simulink library "Ta_Library"  (R2019b)
settings: Solver=VariableStepAuto  StartTime=0.0  StopTime=10.0  RelTol=1e-3
undefined symbols (not defined in the file): AEBSFunctionLib, StateDelayAbortion, TargetClassification
libraries: Mylibrary x5, simulink x1
(part 3 of 3)

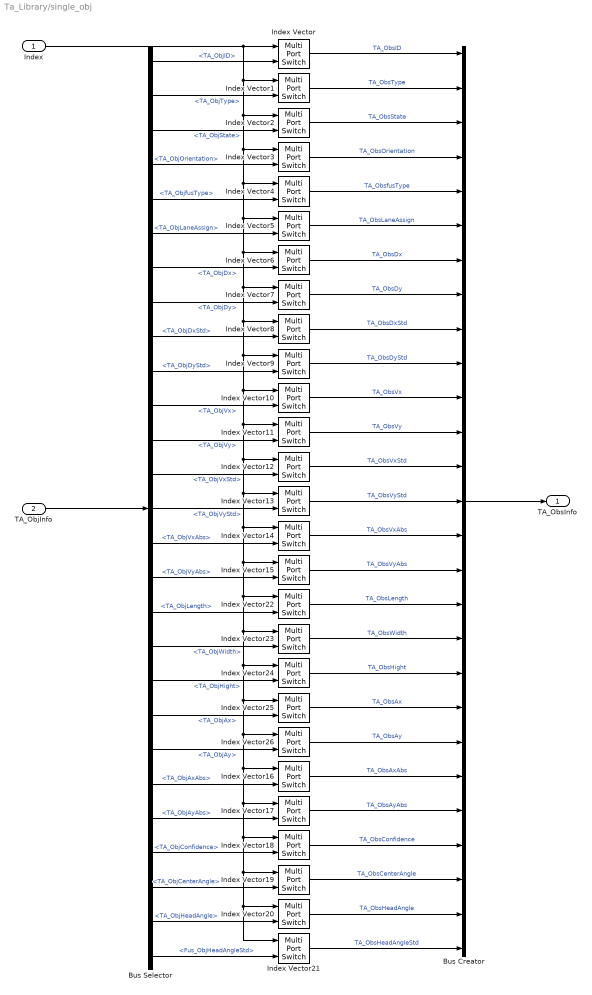
== system Ta_Library/single_obj ==
  Index : Inport
  TA_ObjInfo : Inport  Port=2
  Bus Creator : BusCreator  Inputs=27
  Bus Selector : BusSelector  OutputSignals=TA_ObjID,TA_ObjType,TA_ObjState,TA_ObjOrientation,TA_ObjfusType,TA_ObjLaneAssign,TA_ObjDx,TA_ObjDy,TA_ObjDxStd,TA_ObjDyStd,TA_ObjVx,TA_ObjVy,TA_ObjVxStd,TA_ObjVyStd,TA_ObjVxAbs,TA_ObjVyAbs,TA_ObjLength,TA_ObjWidth,TA_ObjHight,TA_ObjAx,TA_ObjAy,TA_ObjAxAbs,TA_ObjAyAbs,TA_ObjConfidence,TA_ObjCenterAngle,TA_ObjHeadAngle,Fus_ObjHeadAngleStd
  Index Vector{,1..26} (27 alike) : MultiPortSwitch  Inputs=1
  TA_ObsInfo : Outport
  wires:
  TA_ObjInfo/1 -> Bus Selector/1
  Bus Selector/1 -> Index Vector/2  "<TA_ObjID>"
  Index/1 -> Index Vector21/1, Index Vector20/1, Index Vector19/1, Index Vector18/1, Index Vector17/1, Index Vector16/1, Index Vector26/1, Index Vector25/1, Index Vector24/1, Index Vector23/1, Index Vector22/1, Index Vector15/1, Index Vector14/1, Index Vector13/1, Index Vector12/1, Index Vector11/1, Index Vector10/1, Index Vector9/1, Index Vector8/1, Index Vector7/1, Index Vector6/1, Index Vector5/1, Index Vector4/1, Index Vector3/1, Index Vector2/1, Index Vector1/1, Index Vector/1
  Bus Selector/2 -> Index Vector1/2  "<TA_ObjType>"
  Bus Selector/3 -> Index Vector2/2  "<TA_ObjState>"
  Bus Selector/4 -> Index Vector3/2  "<TA_ObjOrientation>"
  Bus Selector/5 -> Index Vector4/2  "<TA_ObjfusType>"
  Bus Selector/6 -> Index Vector5/2  "<TA_ObjLaneAssign>"
  Bus Selector/7 -> Index Vector6/2  "<TA_ObjDx>"
  Bus Selector/8 -> Index Vector7/2  "<TA_ObjDy>"
  Bus Selector/9 -> Index Vector8/2  "<TA_ObjDxStd>"
  Bus Selector/10 -> Index Vector9/2  "<TA_ObjDyStd>"
  Bus Selector/11 -> Index Vector10/2  "<TA_ObjVx>"
  Bus Selector/12 -> Index Vector11/2  "<TA_ObjVy>"
  Bus Selector/13 -> Index Vector12/2  "<TA_ObjVxStd>"
  Bus Selector/14 -> Index Vector13/2  "<TA_ObjVyStd>"
  Bus Selector/15 -> Index Vector14/2  "<TA_ObjVxAbs>"
  Bus Selector/16 -> Index Vector15/2  "<TA_ObjVyAbs>"
  Bus Selector/17 -> Index Vector22/2  "<TA_ObjLength>"
  Bus Selector/18 -> Index Vector23/2  "<TA_ObjWidth>"
  Bus Selector/19 -> Index Vector24/2  "<TA_ObjHight>"
  Bus Selector/20 -> Index Vector25/2  "<TA_ObjAx>"
  Bus Selector/21 -> Index Vector26/2  "<TA_ObjAy>"
  Bus Selector/22 -> Index Vector16/2  "<TA_ObjAxAbs>"
  Bus Selector/23 -> Index Vector17/2  "<TA_ObjAyAbs>"
  Bus Selector/24 -> Index Vector18/2  "<TA_ObjConfidence>"
  Bus Selector/25 -> Index Vector19/2  "<TA_ObjCenterAngle>"
  Bus Selector/26 -> Index Vector20/2  "<TA_ObjHeadAngle>"
  Bus Selector/27 -> Index Vector21/2  "<Fus_ObjHeadAngleStd>"
  Index Vector15/1 -> Bus Creator/16  "TA_ObsVyAbs"
  Index Vector14/1 -> Bus Creator/15  "TA_ObsVxAbs"
  Index Vector22/1 -> Bus Creator/17  "TA_ObsLength"
  Index Vector13/1 -> Bus Creator/14  "TA_ObsVyStd"
  Index Vector23/1 -> Bus Creator/18  "TA_ObsWidth"
  Index Vector12/1 -> Bus Creator/13  "TA_ObsVxStd"
  Index Vector24/1 -> Bus Creator/19  "TA_ObsHight"
  Index Vector11/1 -> Bus Creator/12  "TA_ObsVy"
  Index Vector25/1 -> Bus Creator/20  "TA_ObsAx"
  Index Vector10/1 -> Bus Creator/11  "TA_ObsVx"
  Index Vector26/1 -> Bus Creator/21  "TA_ObsAy"
  Index Vector9/1 -> Bus Creator/10  "TA_ObsDyStd"
  Index Vector16/1 -> Bus Creator/22  "TA_ObsAxAbs"
  Index Vector8/1 -> Bus Creator/9  "TA_ObsDxStd"
  Index Vector17/1 -> Bus Creator/23  "TA_ObsAyAbs"
  Index Vector7/1 -> Bus Creator/8  "TA_ObsDy"
  Index Vector18/1 -> Bus Creator/24  "TA_ObsConfidence"
  Index Vector6/1 -> Bus Creator/7  "TA_ObsDx"
  Index Vector19/1 -> Bus Creator/25  "TA_ObsCenterAngle"
  Index Vector5/1 -> Bus Creator/6  "TA_ObsLaneAssign"
  Index Vector20/1 -> Bus Creator/26  "TA_ObsHeadAngle"
  Index Vector4/1 -> Bus Creator/5  "TA_ObsfusType"
  Index Vector21/1 -> Bus Creator/27  "TA_ObsHeadAngleStd"
  Index Vector3/1 -> Bus Creator/4  "TA_ObsOrientation"
  Index Vector2/1 -> Bus Creator/3  "TA_ObsState"
  Index Vector1/1 -> Bus Creator/2  "TA_ObsType"
  Index Vector/1 -> Bus Creator/1  "TA_ObsID"
  Bus Creator/1 -> TA_ObsInfo/1

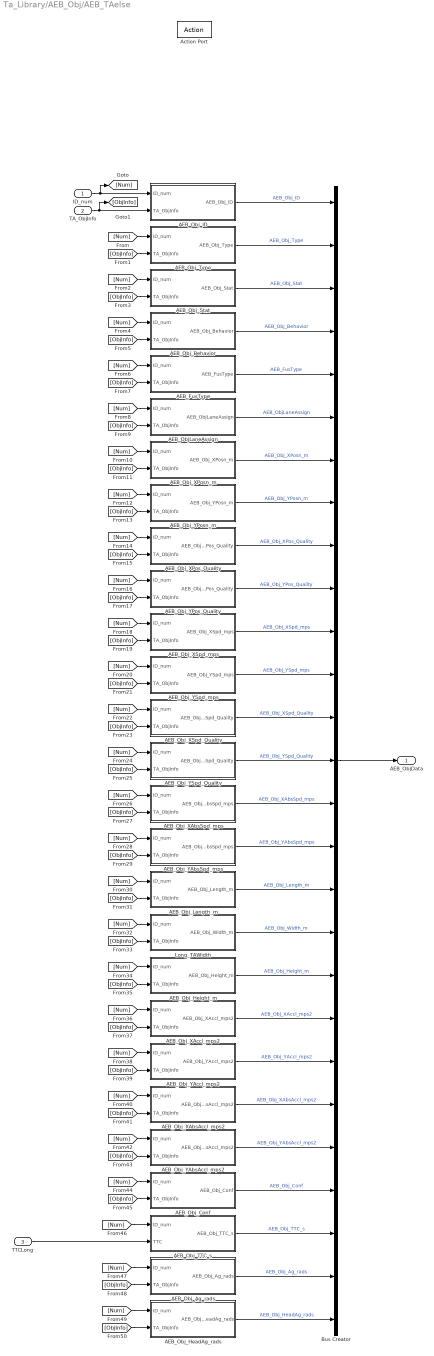
== system Ta_Library/AEB_Obj/AEB_TAelse ==
  ID_num : Inport
  TA_ObjInfo : Inport  Port=2
  TTCLong : Inport  Port=3
  Action Port : ActionPort
  AEB_FusType : Subsystem
  AEB_ObjLaneAssign : Subsystem
  AEB_Obj_Ag_rads : Subsystem
  AEB_Obj_Behavior : Subsystem
  AEB_Obj_Conf : Subsystem
  AEB_Obj_HeadAg_rads : Subsystem
  AEB_Obj_Height_m : Subsystem
  AEB_Obj_ID : Subsystem
  AEB_Obj_Length_m : Subsystem
  AEB_Obj_Stat : Subsystem
  AEB_Obj_TTC_s : Subsystem
  AEB_Obj_Type : Subsystem
  AEB_Obj_XAbsAccl_mps2 : Subsystem
  AEB_Obj_XAbsSpd_mps : Subsystem
  AEB_Obj_XAccl_mps2 : Subsystem
  AEB_Obj_XPos_Quality : Subsystem
  AEB_Obj_XPosn_m : Subsystem
  AEB_Obj_XSpd_Quality : Subsystem
  AEB_Obj_XSpd_mps : Subsystem
  AEB_Obj_YAbsAccl_mps2 : Subsystem
  AEB_Obj_YAbsSpd_mps : Subsystem
  AEB_Obj_YAccl_mps2 : Subsystem
  AEB_Obj_YPos_Quality : Subsystem
  AEB_Obj_YPosn_m : Subsystem
  AEB_Obj_YSpd_Quality : Subsystem
  AEB_Obj_YSpd_mps : Subsystem
  Bus Creator : BusCreator  Inputs=27
  Long_TAWidth : Subsystem
  AEB_ObjData : Outport
  wires:
  Long_TAWidth/1(AEB_Obj_Width_m) -> Bus Creator/18  "AEB_Obj_Width_m"
  AEB_Obj_YSpd_mps/1(AEB_Obj_YSpd_mps) -> Bus Creator/12  "AEB_Obj_YSpd_mps"
  AEB_Obj_XSpd_Quality/1(AEB_Obj_XSpd_Quality) -> Bus Creator/13  "AEB_Obj_XSpd_Quality"
  AEB_Obj_XAbsSpd_mps/1(AEB_Obj_XAbsSpd_mps) -> Bus Creator/15  "AEB_Obj_XAbsSpd_mps"
  AEB_Obj_YSpd_Quality/1(AEB_Obj_YSpd_Quality) -> Bus Creator/14  "AEB_Obj_YSpd_Quality"
  AEB_FusType/1(AEB_FusType) -> Bus Creator/5  "AEB_FusType"
  AEB_ObjLaneAssign/1(AEB_ObjLaneAssign) -> Bus Creator/6  "AEB_ObjLaneAssign"
  AEB_Obj_Length_m/1(AEB_Obj_Length_m) -> Bus Creator/17  "AEB_Obj_Length_m"
  AEB_Obj_XSpd_mps/1(AEB_Obj_XSpd_mps) -> Bus Creator/11  "AEB_Obj_XSpd_mps"
  AEB_Obj_YPos_Quality/1(AEB_Obj_YPos_Quality) -> Bus Creator/10  "AEB_Obj_YPos_Quality"
  AEB_Obj_Type/1(AEB_Obj_Type) -> Bus Creator/2  "AEB_Obj_Type"
  AEB_Obj_YAbsSpd_mps/1(AEB_Obj_YAbsSpd_mps) -> Bus Creator/16  "AEB_Obj_YAbsSpd_mps"
  AEB_Obj_ID/1(AEB_Obj_ID) -> Bus Creator/1  "AEB_Obj_ID"
  AEB_Obj_XPos_Quality/1(AEB_Obj_XPos_Quality) -> Bus Creator/9  "AEB_Obj_XPos_Quality"
  AEB_Obj_Behavior/1(AEB_Obj_Behavior) -> Bus Creator/4  "AEB_Obj_Behavior"
  AEB_Obj_Stat/1(AEB_Obj_Stat) -> Bus Creator/3  "AEB_Obj_Stat"
  AEB_Obj_YPosn_m/1(AEB_Obj_YPosn_m) -> Bus Creator/8  "AEB_Obj_YPosn_m"
  Bus Creator/1 -> AEB_ObjData/1
  AEB_Obj_XPosn_m/1(AEB_Obj_XPosn_m) -> Bus Creator/7  "AEB_Obj_XPosn_m"
  ID_num/1 -> AEB_Obj_ID/1(ID_num), [Num]
  TA_ObjInfo/1 -> [ObjInfo], AEB_Obj_ID/2(TA_ObjInfo)
  [Num] -> AEB_Obj_Type/1(ID_num)
  [ObjInfo] -> AEB_Obj_Type/2(TA_ObjInfo)
  [Num] -> AEB_Obj_Stat/1(ID_num)
  [ObjInfo] -> AEB_Obj_Stat/2(TA_ObjInfo)
  [ObjInfo] -> AEB_Obj_Behavior/2(TA_ObjInfo)
  [Num] -> AEB_Obj_Behavior/1(ID_num)
  [Num] -> AEB_FusType/1(ID_num)
  [ObjInfo] -> AEB_FusType/2(TA_ObjInfo)
  [ObjInfo] -> AEB_ObjLaneAssign/2(TA_ObjInfo)
  [Num] -> AEB_ObjLaneAssign/1(ID_num)
  [Num] -> AEB_Obj_XPosn_m/1(ID_num)
  [ObjInfo] -> AEB_Obj_XPosn_m/2(TA_ObjInfo)
  [ObjInfo] -> AEB_Obj_YPosn_m/2(TA_ObjInfo)
  [Num] -> AEB_Obj_YPosn_m/1(ID_num)
  [Num] -> AEB_Obj_XPos_Quality/1(ID_num)
  [ObjInfo] -> AEB_Obj_XPos_Quality/2(TA_ObjInfo)
  [ObjInfo] -> AEB_Obj_YPos_Quality/2(TA_ObjInfo)
  [Num] -> AEB_Obj_YPos_Quality/1(ID_num)
  [Num] -> AEB_Obj_XSpd_mps/1(ID_num)
  [ObjInfo] -> AEB_Obj_XSpd_mps/2(TA_ObjInfo)
  [ObjInfo] -> AEB_Obj_YSpd_mps/2(TA_ObjInfo)
  [Num] -> AEB_Obj_YSpd_mps/1(ID_num)
  [Num] -> AEB_Obj_XSpd_Quality/1(ID_num)
  [ObjInfo] -> AEB_Obj_XSpd_Quality/2(TA_ObjInfo)
  [ObjInfo] -> AEB_Obj_YSpd_Quality/2(TA_ObjInfo)
  [Num] -> AEB_Obj_YSpd_Quality/1(ID_num)
  [Num] -> AEB_Obj_XAbsSpd_mps/1(ID_num)
  [ObjInfo] -> AEB_Obj_XAbsSpd_mps/2(TA_ObjInfo)
  [ObjInfo] -> AEB_Obj_YAbsSpd_mps/2(TA_ObjInfo)
  [Num] -> AEB_Obj_YAbsSpd_mps/1(ID_num)
  [Num] -> AEB_Obj_Length_m/1(ID_num)
  [ObjInfo] -> AEB_Obj_Length_m/2(TA_ObjInfo)
  [ObjInfo] -> Long_TAWidth/2(TA_ObjInfo)
  [Num] -> Long_TAWidth/1(ID_num)
  [Num] -> AEB_Obj_Height_m/1(ID_num)
  [ObjInfo] -> AEB_Obj_Height_m/2(TA_ObjInfo)
  AEB_Obj_Height_m/1(AEB_Obj_Height_m) -> Bus Creator/19  "AEB_Obj_Height_m"
  [ObjInfo] -> AEB_Obj_XAccl_mps2/2(TA_ObjInfo)
  [Num] -> AEB_Obj_XAccl_mps2/1(ID_num)
  [Num] -> AEB_Obj_YAccl_mps2/1(ID_num)
  [ObjInfo] -> AEB_Obj_YAccl_mps2/2(TA_ObjInfo)
  [ObjInfo] -> AEB_Obj_YAbsAccl_mps2/2(TA_ObjInfo)
  [Num] -> AEB_Obj_YAbsAccl_mps2/1(ID_num)
  [Num] -> AEB_Obj_XAbsAccl_mps2/1(ID_num)
  [ObjInfo] -> AEB_Obj_XAbsAccl_mps2/2(TA_ObjInfo)
  [Num] -> AEB_Obj_Conf/1(ID_num)
  [ObjInfo] -> AEB_Obj_Conf/2(TA_ObjInfo)
  [Num] -> AEB_Obj_TTC_s/1(ID_num)
  TTCLong/1 -> AEB_Obj_TTC_s/2(TTC)
  [ObjInfo] -> AEB_Obj_Ag_rads/2(TA_ObjInfo)
  [Num] -> AEB_Obj_Ag_rads/1(ID_num)
  [Num] -> AEB_Obj_HeadAg_rads/1(ID_num)
  [ObjInfo] -> AEB_Obj_HeadAg_rads/2(TA_ObjInfo)
  AEB_Obj_XAccl_mps2/1(AEB_Obj_XAccl_mps2) -> Bus Creator/20  "AEB_Obj_XAccl_mps2"
  AEB_Obj_YAccl_mps2/1(AEB_Obj_YAccl_mps2) -> Bus Creator/21  "AEB_Obj_YAccl_mps2"
  AEB_Obj_XAbsAccl_mps2/1(AEB_Obj_XAbsAccl_mps2) -> Bus Creator/22  "AEB_Obj_XAbsAccl_mps2"
  AEB_Obj_YAbsAccl_mps2/1(AEB_Obj_YAbsAccl_mps2) -> Bus Creator/23  "AEB_Obj_YAbsAccl_mps2"
  AEB_Obj_Conf/1(AEB_Obj_Conf) -> Bus Creator/24  "AEB_Obj_Conf"
  AEB_Obj_TTC_s/1(AEB_Obj_TTC_s) -> Bus Creator/25  "AEB_Obj_TTC_s"
  AEB_Obj_Ag_rads/1(AEB_Obj_Ag_rads) -> Bus Creator/26  "AEB_Obj_Ag_rads"
  AEB_Obj_HeadAg_rads/1(AEB_Obj_HeadAg_rads) -> Bus Creator/27  "AEB_Obj_HeadAg_rads"

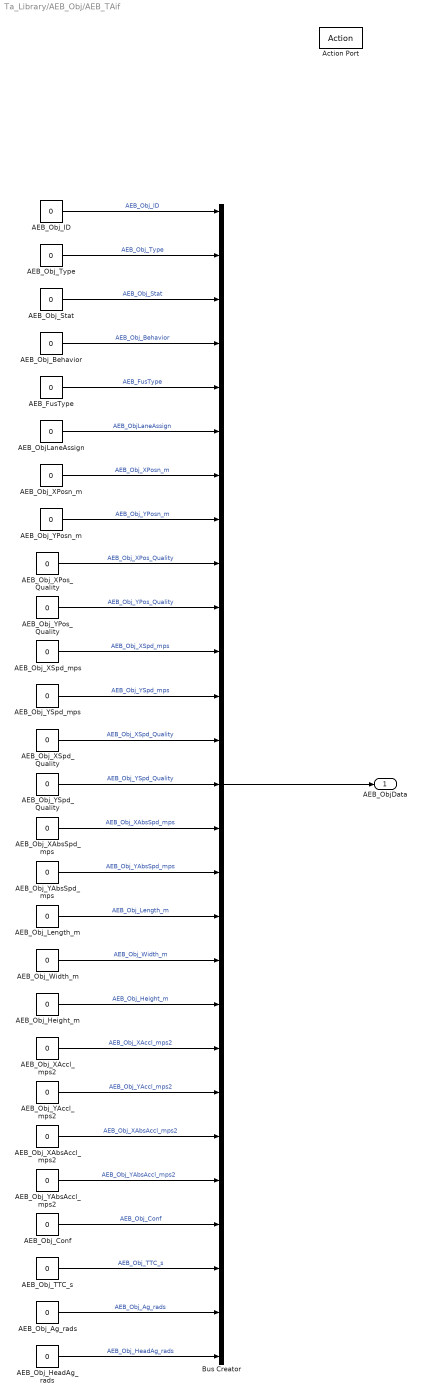
== system Ta_Library/AEB_Obj/AEB_TAif ==
  Action Port : ActionPort
  AEB_FusType : Constant  Value=0  OutDataTypeStr=uint8
  AEB_ObjLaneAssign : Constant  Value=0  OutDataTypeStr=uint8
  AEB_Obj_Ag_rads : Constant  Value=0  OutDataTypeStr=single
  AEB_Obj_Behavior : Constant  Value=0  OutDataTypeStr=uint8
  AEB_Obj_Conf : Constant  Value=0  OutDataTypeStr=uint8
  AEB_Obj_HeadAg_rads : Constant  Value=0  OutDataTypeStr=single
  AEB_Obj_Height_m : Constant  Value=0  OutDataTypeStr=single
  AEB_Obj_ID : Constant  Value=0  OutDataTypeStr=uint8
  AEB_Obj_Length_m : Constant  Value=0  OutDataTypeStr=single
  AEB_Obj_Stat : Constant  Value=0  OutDataTypeStr=uint8
  AEB_Obj_TTC_s : Constant  Value=0  OutDataTypeStr=single
  AEB_Obj_Type : Constant  Value=0  OutDataTypeStr=uint8
  AEB_Obj_Width_m : Constant  Value=0  OutDataTypeStr=single
  AEB_Obj_XAbsAccl_mps2 : Constant  Value=0  OutDataTypeStr=single
  AEB_Obj_XAbsSpd_mps : Constant  Value=0  OutDataTypeStr=single
  AEB_Obj_XAccl_mps2 : Constant  Value=0  OutDataTypeStr=single
  AEB_Obj_XPos_Quality : Constant  Value=0  OutDataTypeStr=single
  AEB_Obj_XPosn_m : Constant  Value=0  OutDataTypeStr=single
  AEB_Obj_XSpd_Quality : Constant  Value=0  OutDataTypeStr=single
  AEB_Obj_XSpd_mps : Constant  Value=0  OutDataTypeStr=single
  AEB_Obj_YAbsAccl_mps2 : Constant  Value=0  OutDataTypeStr=single
  AEB_Obj_YAbsSpd_mps : Constant  Value=0  OutDataTypeStr=single
  AEB_Obj_YAccl_mps2 : Constant  Value=0  OutDataTypeStr=single
  AEB_Obj_YPos_Quality : Constant  Value=0  OutDataTypeStr=single
  AEB_Obj_YPosn_m : Constant  Value=0  OutDataTypeStr=single
  AEB_Obj_YSpd_Quality : Constant  Value=0  OutDataTypeStr=single
  AEB_Obj_YSpd_mps : Constant  Value=0  OutDataTypeStr=single
  Bus Creator : BusCreator  Inputs=27
  AEB_ObjData : Outport
  wires:
  AEB_Obj_ID/1 -> Bus Creator/1  "AEB_Obj_ID"
  AEB_Obj_Type/1 -> Bus Creator/2  "AEB_Obj_Type"
  AEB_Obj_Stat/1 -> Bus Creator/3  "AEB_Obj_Stat"
  AEB_Obj_Behavior/1 -> Bus Creator/4  "AEB_Obj_Behavior"
  AEB_FusType/1 -> Bus Creator/5  "AEB_FusType"
  AEB_ObjLaneAssign/1 -> Bus Creator/6  "AEB_ObjLaneAssign"
  AEB_Obj_XPosn_m/1 -> Bus Creator/7  "AEB_Obj_XPosn_m"
  AEB_Obj_YPosn_m/1 -> Bus Creator/8  "AEB_Obj_YPosn_m"
  AEB_Obj_XPos_Quality/1 -> Bus Creator/9  "AEB_Obj_XPos_Quality"
  AEB_Obj_YPos_Quality/1 -> Bus Creator/10  "AEB_Obj_YPos_Quality"
  AEB_Obj_XSpd_mps/1 -> Bus Creator/11  "AEB_Obj_XSpd_mps"
  AEB_Obj_YSpd_mps/1 -> Bus Creator/12  "AEB_Obj_YSpd_mps"
  AEB_Obj_XSpd_Quality/1 -> Bus Creator/13  "AEB_Obj_XSpd_Quality"
  AEB_Obj_YSpd_Quality/1 -> Bus Creator/14  "AEB_Obj_YSpd_Quality"
  AEB_Obj_XAbsSpd_mps/1 -> Bus Creator/15  "AEB_Obj_XAbsSpd_mps"
  AEB_Obj_YAbsSpd_mps/1 -> Bus Creator/16  "AEB_Obj_YAbsSpd_mps"
  AEB_Obj_Length_m/1 -> Bus Creator/17  "AEB_Obj_Length_m"
  AEB_Obj_Width_m/1 -> Bus Creator/18  "AEB_Obj_Width_m"
  AEB_Obj_Height_m/1 -> Bus Creator/19  "AEB_Obj_Height_m"
  Bus Creator/1 -> AEB_ObjData/1
  AEB_Obj_XAbsAccl_mps2/1 -> Bus Creator/22  "AEB_Obj_XAbsAccl_mps2"
  AEB_Obj_YAbsAccl_mps2/1 -> Bus Creator/23  "AEB_Obj_YAbsAccl_mps2"
  AEB_Obj_XAccl_mps2/1 -> Bus Creator/20  "AEB_Obj_XAccl_mps2"
  AEB_Obj_TTC_s/1 -> Bus Creator/25  "AEB_Obj_TTC_s"
  AEB_Obj_Ag_rads/1 -> Bus Creator/26  "AEB_Obj_Ag_rads"
  AEB_Obj_HeadAg_rads/1 -> Bus Creator/27  "AEB_Obj_HeadAg_rads"
  AEB_Obj_YAccl_mps2/1 -> Bus Creator/21  "AEB_Obj_YAccl_mps2"
  AEB_Obj_Conf/1 -> Bus Creator/24  "AEB_Obj_Conf"

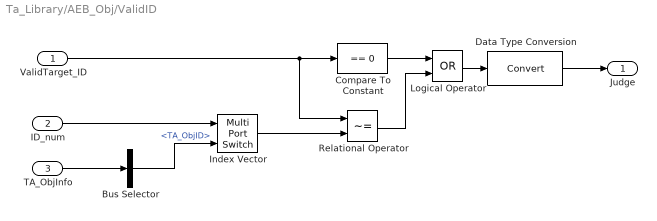
== system Ta_Library/AEB_Obj/ValidID ==
  ValidTarget_ID : Inport
  ID_num : Inport  Port=2
  TA_ObjInfo : Inport  Port=3
  Bus Selector : BusSelector  OutputSignals=TA_ObjInfo.TA_ObjID
  Compare To Constant : simulink/Logic and Bit Operations/Compare To Constant  relop===  const=0  OutDataTypeStr=boolean
  Data Type Conversion : DataTypeConversion
  Index Vector : MultiPortSwitch  Inputs=1
  Logical Operator : Logic  Operator=OR  AllPortsSameDT=off  OutDataTypeStr=boolean
  Relational Operator : RelationalOperator  Operator=~=  OutDataTypeStr=boolean  RndMeth=Simplest
  Judge : Outport
  wires:
  ValidTarget_ID/1 -> Relational Operator/1, Compare To Constant/1
  Data Type Conversion/1 -> Judge/1
  ID_num/1 -> Index Vector/1
  TA_ObjInfo/1 -> Bus Selector/1
  Bus Selector/1 -> Index Vector/2  "<TA_ObjID>"
  Index Vector/1 -> Relational Operator/2
  Compare To Constant/1 -> Logical Operator/1
  Relational Operator/1 -> Logical Operator/2
  Logical Operator/1 -> Data Type Conversion/1

== system Ta_Library/AEB_Obj/AEB_TAelse/AEB_FusType ==
  ID_num : Inport
  TA_ObjInfo : Inport  Port=2
  Bus Selector : BusSelector  OutputSignals=TA_ObjInfo.TA_ObjfusType
  Index Vector : MultiPortSwitch  Inputs=1
  AEB_FusType : Outport
  wires:
  TA_ObjInfo/1 -> Bus Selector/1
  Bus Selector/1 -> Index Vector/2  "<TA_ObjfusType>"
  ID_num/1 -> Index Vector/1
  Index Vector/1 -> AEB_FusType/1

== system Ta_Library/AEB_Obj/AEB_TAelse/AEB_ObjLaneAssign ==
  ID_num : Inport
  TA_ObjInfo : Inport  Port=2
  Bus Selector : BusSelector  OutputSignals=TA_ObjInfo.TA_ObjLaneAssign
  Index Vector : MultiPortSwitch  Inputs=1
  AEB_ObjLaneAssign : Outport
  wires:
  Index Vector/1 -> AEB_ObjLaneAssign/1
  ID_num/1 -> Index Vector/1
  Bus Selector/1 -> Index Vector/2  "<TA_ObjLaneAssign>"
  TA_ObjInfo/1 -> Bus Selector/1

== system Ta_Library/AEB_Obj/AEB_TAelse/AEB_Obj_Ag_rads ==
  ID_num : Inport
  TA_ObjInfo : Inport  Port=2
  Bus Selector : BusSelector  OutputSignals=TA_ObjInfo.TA_ObjCenterAngle
  Index Vector : MultiPortSwitch  Inputs=1
  AEB_Obj_Ag_rads : Outport
  wires:
  Index Vector/1 -> AEB_Obj_Ag_rads/1
  ID_num/1 -> Index Vector/1
  Bus Selector/1 -> Index Vector/2  "<TA_ObjCenterAngle>"
  TA_ObjInfo/1 -> Bus Selector/1

== system Ta_Library/AEB_Obj/AEB_TAelse/AEB_Obj_Behavior ==
  ID_num : Inport
  TA_ObjInfo : Inport  Port=2
  Bus Selector : BusSelector  OutputSignals=TA_ObjInfo.TA_ObjOrientation
  Index Vector : MultiPortSwitch  Inputs=1
  AEB_Obj_Behavior : Outport
  wires:
  Index Vector/1 -> AEB_Obj_Behavior/1
  ID_num/1 -> Index Vector/1
  Bus Selector/1 -> Index Vector/2  "<TA_ObjOrientation>"
  TA_ObjInfo/1 -> Bus Selector/1

== system Ta_Library/AEB_Obj/AEB_TAelse/AEB_Obj_Conf ==
  ID_num : Inport
  TA_ObjInfo : Inport  Port=2
  Bus Selector : BusSelector  OutputSignals=TA_ObjInfo.TA_ObjConfidence
  Index Vector : MultiPortSwitch  Inputs=1
  AEB_Obj_Conf : Outport
  wires:
  TA_ObjInfo/1 -> Bus Selector/1
  Bus Selector/1 -> Index Vector/2  "<TA_ObjConfidence>"
  ID_num/1 -> Index Vector/1
  Index Vector/1 -> AEB_Obj_Conf/1

== system Ta_Library/AEB_Obj/AEB_TAelse/AEB_Obj_HeadAg_rads ==
  ID_num : Inport
  TA_ObjInfo : Inport  Port=2
  Bus Selector : BusSelector  OutputSignals=TA_ObjInfo.TA_ObjHeadAngle
  Index Vector : MultiPortSwitch  Inputs=1
  AEB_Obj_HeadAg_rads : Outport
  wires:
  TA_ObjInfo/1 -> Bus Selector/1
  Bus Selector/1 -> Index Vector/2  "<TA_ObjHeadAngle>"
  ID_num/1 -> Index Vector/1
  Index Vector/1 -> AEB_Obj_HeadAg_rads/1

== system Ta_Library/AEB_Obj/AEB_TAelse/AEB_Obj_Height_m ==
  ID_num : Inport
  TA_ObjInfo : Inport  Port=2
  Bus Selector : BusSelector  OutputSignals=TA_ObjInfo.TA_ObjHight
  Index Vector : MultiPortSwitch  Inputs=1
  AEB_Obj_Height_m : Outport
  wires:
  TA_ObjInfo/1 -> Bus Selector/1
  Bus Selector/1 -> Index Vector/2  "<TA_ObjHight>"
  ID_num/1 -> Index Vector/1
  Index Vector/1 -> AEB_Obj_Height_m/1

== system Ta_Library/AEB_Obj/AEB_TAelse/AEB_Obj_ID ==
  ID_num : Inport
  TA_ObjInfo : Inport  Port=2
  Bus Selector : BusSelector  OutputSignals=TA_ObjInfo.TA_ObjID
  Index Vector : MultiPortSwitch  Inputs=1
  AEB_Obj_ID : Outport
  wires:
  TA_ObjInfo/1 -> Bus Selector/1
  Bus Selector/1 -> Index Vector/2  "<TA_ObjID>"
  ID_num/1 -> Index Vector/1
  Index Vector/1 -> AEB_Obj_ID/1

== system Ta_Library/AEB_Obj/AEB_TAelse/AEB_Obj_Length_m ==
  ID_num : Inport
  TA_ObjInfo : Inport  Port=2
  Bus Selector : BusSelector  OutputSignals=TA_ObjInfo.TA_ObjLength
  Index Vector : MultiPortSwitch  Inputs=1
  AEB_Obj_Length_m : Outport
  wires:
  TA_ObjInfo/1 -> Bus Selector/1
  Bus Selector/1 -> Index Vector/2  "<TA_ObjLength>"
  ID_num/1 -> Index Vector/1
  Index Vector/1 -> AEB_Obj_Length_m/1

== system Ta_Library/AEB_Obj/AEB_TAelse/AEB_Obj_Stat ==
  ID_num : Inport
  TA_ObjInfo : Inport  Port=2
  Bus Selector : BusSelector  OutputSignals=TA_ObjInfo.TA_ObjState
  Index Vector : MultiPortSwitch  Inputs=1
  AEB_Obj_Stat : Outport
  wires:
  TA_ObjInfo/1 -> Bus Selector/1
  Bus Selector/1 -> Index Vector/2  "<TA_ObjState>"
  ID_num/1 -> Index Vector/1
  Index Vector/1 -> AEB_Obj_Stat/1

== system Ta_Library/AEB_Obj/AEB_TAelse/AEB_Obj_TTC_s ==
  ID_num : Inport
  TTC : Inport  Port=2
  Signal Conversion : SignalConversion  OverrideOpt=off
  Terminator : Terminator
  AEB_Obj_TTC_s : Outport
  wires:
  Signal Conversion/1 -> AEB_Obj_TTC_s/1
  ID_num/1 -> Terminator/1
  TTC/1 -> Signal Conversion/1

== system Ta_Library/AEB_Obj/AEB_TAelse/AEB_Obj_Type ==
  ID_num : Inport
  TA_ObjInfo : Inport  Port=2
  Bus Selector : BusSelector  OutputSignals=TA_ObjInfo.TA_ObjType
  Index Vector : MultiPortSwitch  Inputs=1
  AEB_Obj_Type : Outport
  wires:
  Index Vector/1 -> AEB_Obj_Type/1
  ID_num/1 -> Index Vector/1
  Bus Selector/1 -> Index Vector/2  "<TA_ObjType>"
  TA_ObjInfo/1 -> Bus Selector/1

== system Ta_Library/AEB_Obj/AEB_TAelse/AEB_Obj_XAbsAccl_mps2 ==
  ID_num : Inport
  TA_ObjInfo : Inport  Port=2
  Bus Selector : BusSelector  OutputSignals=TA_ObjInfo.TA_ObjAxAbs
  Index Vector : MultiPortSwitch  Inputs=1
  AEB_Obj_XAbsAccl_mps2 : Outport
  wires:
  TA_ObjInfo/1 -> Bus Selector/1
  Bus Selector/1 -> Index Vector/2  "<TA_ObjAxAbs>"
  ID_num/1 -> Index Vector/1
  Index Vector/1 -> AEB_Obj_XAbsAccl_mps2/1

== system Ta_Library/AEB_Obj/AEB_TAelse/AEB_Obj_XAbsSpd_mps ==
  ID_num : Inport
  TA_ObjInfo : Inport  Port=2
  Bus Selector : BusSelector  OutputSignals=TA_ObjInfo.TA_ObjVxAbs
  Index Vector : MultiPortSwitch  Inputs=1
  AEB_Obj_XAbsSpd_mps : Outport
  wires:
  TA_ObjInfo/1 -> Bus Selector/1
  Bus Selector/1 -> Index Vector/2  "<TA_ObjVxAbs>"
  ID_num/1 -> Index Vector/1
  Index Vector/1 -> AEB_Obj_XAbsSpd_mps/1

== system Ta_Library/AEB_Obj/AEB_TAelse/AEB_Obj_XAccl_mps2 ==
  ID_num : Inport
  TA_ObjInfo : Inport  Port=2
  Bus Selector : BusSelector  OutputSignals=TA_ObjInfo.TA_ObjAx
  Index Vector : MultiPortSwitch  Inputs=1
  AEB_Obj_XAccl_mps2 : Outport
  wires:
  Index Vector/1 -> AEB_Obj_XAccl_mps2/1
  ID_num/1 -> Index Vector/1
  Bus Selector/1 -> Index Vector/2  "<TA_ObjAx>"
  TA_ObjInfo/1 -> Bus Selector/1

== system Ta_Library/AEB_Obj/AEB_TAelse/AEB_Obj_XPos_Quality ==
  ID_num : Inport
  TA_ObjInfo : Inport  Port=2
  Bus Selector : BusSelector  OutputSignals=TA_ObjInfo.TA_ObjDxStd
  Index Vector : MultiPortSwitch  Inputs=1
  AEB_Obj_XPos_Quality : Outport
  wires:
  TA_ObjInfo/1 -> Bus Selector/1
  Bus Selector/1 -> Index Vector/2  "<TA_ObjDxStd>"
  ID_num/1 -> Index Vector/1
  Index Vector/1 -> AEB_Obj_XPos_Quality/1

== system Ta_Library/AEB_Obj/AEB_TAelse/AEB_Obj_XPosn_m ==
  ID_num : Inport
  TA_ObjInfo : Inport  Port=2
  Bus Selector : BusSelector  OutputSignals=TA_ObjInfo.TA_ObjDx
  Index Vector : MultiPortSwitch  Inputs=1
  AEB_Obj_XPosn_m : Outport
  wires:
  TA_ObjInfo/1 -> Bus Selector/1
  Bus Selector/1 -> Index Vector/2  "<TA_ObjDx>"
  ID_num/1 -> Index Vector/1
  Index Vector/1 -> AEB_Obj_XPosn_m/1

== system Ta_Library/AEB_Obj/AEB_TAelse/AEB_Obj_XSpd_Quality ==
  ID_num : Inport
  TA_ObjInfo : Inport  Port=2
  Bus Selector : BusSelector  OutputSignals=TA_ObjInfo.TA_ObjVxStd
  Index Vector : MultiPortSwitch  Inputs=1
  AEB_Obj_XSpd_Quality : Outport
  wires:
  TA_ObjInfo/1 -> Bus Selector/1
  Bus Selector/1 -> Index Vector/2  "<TA_ObjVxStd>"
  ID_num/1 -> Index Vector/1
  Index Vector/1 -> AEB_Obj_XSpd_Quality/1

== system Ta_Library/AEB_Obj/AEB_TAelse/AEB_Obj_XSpd_mps ==
  ID_num : Inport
  TA_ObjInfo : Inport  Port=2
  Bus Selector : BusSelector  OutputSignals=TA_ObjInfo.TA_ObjVx
  Index Vector : MultiPortSwitch  Inputs=1
  AEB_Obj_XSpd_mps : Outport
  wires:
  TA_ObjInfo/1 -> Bus Selector/1
  Bus Selector/1 -> Index Vector/2  "<TA_ObjVx>"
  ID_num/1 -> Index Vector/1
  Index Vector/1 -> AEB_Obj_XSpd_mps/1

== system Ta_Library/AEB_Obj/AEB_TAelse/AEB_Obj_YAbsAccl_mps2 ==
  ID_num : Inport
  TA_ObjInfo : Inport  Port=2
  Bus Selector : BusSelector  OutputSignals=TA_ObjInfo.TA_ObjAyAbs
  Index Vector : MultiPortSwitch  Inputs=1
  AEB_Obj_YAbsAccl_mps2 : Outport
  wires:
  Index Vector/1 -> AEB_Obj_YAbsAccl_mps2/1
  ID_num/1 -> Index Vector/1
  Bus Selector/1 -> Index Vector/2  "<TA_ObjAyAbs>"
  TA_ObjInfo/1 -> Bus Selector/1

== system Ta_Library/AEB_Obj/AEB_TAelse/AEB_Obj_YAbsSpd_mps ==
  ID_num : Inport
  TA_ObjInfo : Inport  Port=2
  Bus Selector : BusSelector  OutputSignals=TA_ObjInfo.TA_ObjVyAbs
  Index Vector : MultiPortSwitch  Inputs=1
  AEB_Obj_YAbsSpd_mps : Outport
  wires:
  Index Vector/1 -> AEB_Obj_YAbsSpd_mps/1
  ID_num/1 -> Index Vector/1
  Bus Selector/1 -> Index Vector/2  "<TA_ObjVyAbs>"
  TA_ObjInfo/1 -> Bus Selector/1

== system Ta_Library/AEB_Obj/AEB_TAelse/AEB_Obj_YAccl_mps2 ==
  ID_num : Inport
  TA_ObjInfo : Inport  Port=2
  Bus Selector : BusSelector  OutputSignals=TA_ObjInfo.TA_ObjAyAbs
  Index Vector : MultiPortSwitch  Inputs=1
  AEB_Obj_YAccl_mps2 : Outport
  wires:
  TA_ObjInfo/1 -> Bus Selector/1
  Bus Selector/1 -> Index Vector/2  "<TA_ObjAyAbs>"
  ID_num/1 -> Index Vector/1
  Index Vector/1 -> AEB_Obj_YAccl_mps2/1

== system Ta_Library/AEB_Obj/AEB_TAelse/AEB_Obj_YPos_Quality ==
  ID_num : Inport
  TA_ObjInfo : Inport  Port=2
  Bus Selector : BusSelector  OutputSignals=TA_ObjInfo.TA_ObjDyStd
  Index Vector : MultiPortSwitch  Inputs=1
  AEB_Obj_YPos_Quality : Outport
  wires:
  Index Vector/1 -> AEB_Obj_YPos_Quality/1
  ID_num/1 -> Index Vector/1
  Bus Selector/1 -> Index Vector/2  "<TA_ObjDyStd>"
  TA_ObjInfo/1 -> Bus Selector/1

== system Ta_Library/AEB_Obj/AEB_TAelse/AEB_Obj_YPosn_m ==
  ID_num : Inport
  TA_ObjInfo : Inport  Port=2
  Bus Selector : BusSelector  OutputSignals=TA_ObjInfo.TA_ObjDy
  Index Vector : MultiPortSwitch  Inputs=1
  AEB_Obj_YPosn_m : Outport
  wires:
  Index Vector/1 -> AEB_Obj_YPosn_m/1
  ID_num/1 -> Index Vector/1
  Bus Selector/1 -> Index Vector/2  "<TA_ObjDy>"
  TA_ObjInfo/1 -> Bus Selector/1

== system Ta_Library/AEB_Obj/AEB_TAelse/AEB_Obj_YSpd_Quality ==
  ID_num : Inport
  TA_ObjInfo : Inport  Port=2
  Bus Selector : BusSelector  OutputSignals=TA_ObjInfo.TA_ObjVyStd
  Index Vector : MultiPortSwitch  Inputs=1
  AEB_Obj_YSpd_Quality : Outport
  wires:
  Index Vector/1 -> AEB_Obj_YSpd_Quality/1
  ID_num/1 -> Index Vector/1
  Bus Selector/1 -> Index Vector/2  "<TA_ObjVyStd>"
  TA_ObjInfo/1 -> Bus Selector/1

== system Ta_Library/AEB_Obj/AEB_TAelse/AEB_Obj_YSpd_mps ==
  ID_num : Inport
  TA_ObjInfo : Inport  Port=2
  Bus Selector : BusSelector  OutputSignals=TA_ObjInfo.TA_ObjVy
  Index Vector : MultiPortSwitch  Inputs=1
  AEB_Obj_YSpd_mps : Outport
  wires:
  Index Vector/1 -> AEB_Obj_YSpd_mps/1
  ID_num/1 -> Index Vector/1
  Bus Selector/1 -> Index Vector/2  "<TA_ObjVy>"
  TA_ObjInfo/1 -> Bus Selector/1

== system Ta_Library/AEB_Obj/AEB_TAelse/Long_TAWidth ==
  ID_num : Inport
  TA_ObjInfo : Inport  Port=2
  Bus Selector : BusSelector  OutputSignals=TA_ObjInfo.TA_ObjWidth
  Index Vector : MultiPortSwitch  Inputs=1
  AEB_Obj_Width_m : Outport
  wires:
  Index Vector/1 -> AEB_Obj_Width_m/1
  ID_num/1 -> Index Vector/1
  Bus Selector/1 -> Index Vector/2  "<TA_ObjWidth>"
  TA_ObjInfo/1 -> Bus Selector/1

== stateflow chart Ta_Library/AccReleventSuppCondStateDelayAbortion/StateDelayAbortion ==
  state NormalState
    en:
    stateOut = state;
    CNTimeCounterMAX = 256;
    du:
    stateOut = state;
  state CounterState
    en:
    timeSinceLastState = 0;
    du:
    timeSinceLastState +=  Ts;
    CounterStateFunc();
  state CounterStateFunc [function]
    (default) -> (junction 70)
    (junction 70) -> (junction 62) [order 1] : [timeSinceLastState > CNTimeCounterMAX]
    (junction 70) -> (junction 69) [order 2] : %do nothing
    (junction 62) -> (junction 61) : {
        | 	timeSinceLastState = CNTimeCounterMAX;
        | }
    (junction 61) -> (junction 69)
    (junction 69) -> (junction 68)
    (junction 68) -> (junction 60) [order 1] : [timeSinceLastState < stateProlongationTime]
    (junction 68) -> (junction 66) [order 2] : {
        | 	stateOut = false;
        | }
    (junction 60) -> (junction 67) : {
        | 	stateOut = true;
        | }
    (junction 67) -> (junction 66)
    (junction 66) -> (junction 56)
  (default) -> NormalState
  NormalState -> CounterState : [stateK1 == true &&...
      | state == false]
  CounterState -> NormalState : [timeSinceLastState > stateProlongationTime]
  data: state input; stateK1 input; stateProlongationTime input; timeSinceLastState output double; stateOut output boolean; Ts input; CNTimeCounterMAX local double

== stateflow chart Ta_Library/StrReleventSuppCondDelayAbortion/StateDelayAbortion ==
  state NormalState
    en:
    stateOut = state;
    CNTimeCounterMAX = 256;
    du:
    stateOut = state;
  state CounterState
    en:
    timeSinceLastState = 0;
    du:
    timeSinceLastState +=  Ts;
    CounterStateFunc();
  state CounterStateFunc [function]
    (default) -> (junction 70)
    (junction 70) -> (junction 62) [order 1] : [timeSinceLastState > CNTimeCounterMAX]
    (junction 70) -> (junction 69) [order 2] : %do nothing
    (junction 62) -> (junction 61) : {
        | 	timeSinceLastState = CNTimeCounterMAX;
        | }
    (junction 61) -> (junction 69)
    (junction 69) -> (junction 68)
    (junction 68) -> (junction 60) [order 1] : [timeSinceLastState < stateProlongationTime]
    (junction 68) -> (junction 66) [order 2] : {
        | 	stateOut = false;
        | }
    (junction 60) -> (junction 67) : {
        | 	stateOut = true;
        | }
    (junction 67) -> (junction 66)
    (junction 66) -> (junction 56)
  (default) -> NormalState
  NormalState -> CounterState : [stateK1 == true &&...
      | state == false]
  CounterState -> NormalState : [timeSinceLastState > stateProlongationTime]
  data: state input; stateK1 input; stateProlongationTime input; timeSinceLastState output double; stateOut output boolean; Ts input; CNTimeCounterMAX local double
